simulink model "rc3"  (R2018a)
settings: Solver=FixedStepAuto  StartTime=0.0  StopTime=10  FixedStep=1e-5  RelTol=1e-3
settings Model: Creator=user  LastModifiedBy=user

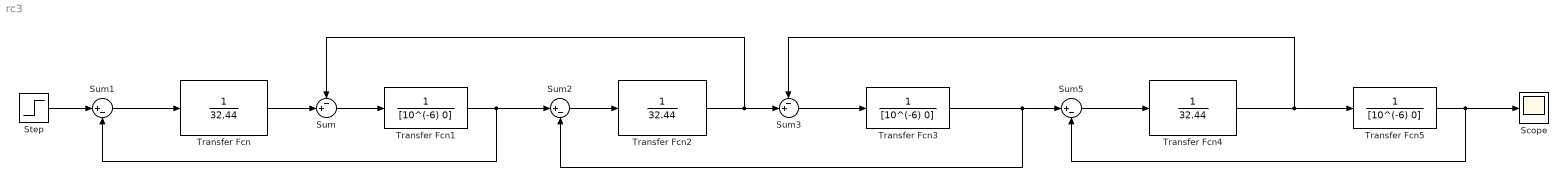
== system rc3 ==
  Scope : Scope
  Step : Step  SampleTime=0
  Sum : Sum  Inputs=-+|
  Sum1 : Sum  Inputs=|+-
  Sum2 : Sum  Inputs=|+-
  Sum3 : Sum  Inputs=-+|
  Sum5 : Sum  Inputs=|+-
  Transfer Fcn : TransferFcn  Denominator=[32.44]
  Transfer Fcn1 : TransferFcn  Denominator=[10^(-6) 0]
  Transfer Fcn2 : TransferFcn  Denominator=[32.44]
  Transfer Fcn3 : TransferFcn  Denominator=[10^(-6) 0]
  Transfer Fcn4 : TransferFcn  Denominator=[32.44]
  Transfer Fcn5 : TransferFcn  Denominator=[10^(-6) 0]
  wires:
  Sum1/1 -> Transfer Fcn/1
  Transfer Fcn1/1 -> Sum2/1, Sum1/2
  Step/1 -> Sum1/1
  Transfer Fcn/1 -> Sum/2
  Sum/1 -> Transfer Fcn1/1
  Sum2/1 -> Transfer Fcn2/1
  Transfer Fcn2/1 -> Sum3/2, Sum/1
  Transfer Fcn3/1 -> Sum5/1, Sum2/2
  Sum3/1 -> Transfer Fcn3/1
  Transfer Fcn5/1 -> Scope/1, Sum5/2
  Sum5/1 -> Transfer Fcn4/1
  Transfer Fcn4/1 -> Sum3/1, Transfer Fcn5/1
